simulink model "s1"  (Simulink 2.00)
settings: Solver=ode113  StartTime=0.0  StopTime=tstop  MaxStep=1e-3  RelTol=1e-6  AbsTol=1e-5
values from neighbouring files (symbols this model uses):
  Domega = 0    [P1HP.M]    (also in PSPH.M)
  H = J*wbm*wbm/(2*Sb)    (= 2.36870505626)    [P1HP.M]    (also in PSPH.M = 1.39074103839)
  Psidso = 0    [M1.M]    (also in M4.M; M4STP.M; M5.M)
  Psipdro = 0    [M1.M]    (also in M4.M; M4STP.M; M5.M; M6.M)
  Psipqro = 0    [M1.M]    (also in M4.M = Vm; M4STP.M = Vm; M5.M; M6.M)
  Psiqso = 0    [M1.M]    (also in M4.M = Vm; M4STP.M = Vm; M5.M; M6.M)
  rpr = 1.99    [P1HP.M]    (also in PSPH.M = 4.12)
  rs = 3.35    [P1HP.M]
  Tfactor = (3*P)/(4*wb)    (= 0.00795774715459)    [P1HP.M]    (also in PSPH.M = 0.00530516476973)
  tmech_time = [0 0.8 0.8 1.2 1.2 1.6 1.6 tstop]    [M1.M]    (also in M6.M = [0 1.5 1.5 1.75 1.75 2.0 2.0 2.25 2.25 2.5])
  tmech_value = [0 0 -0.5 -0.5 -1. -1. -0.5 -0.5]*Tb    [M1.M]    (also in M6.M = [0 0 -Tb -Tb -Tb/2 -Tb/2 -Tb -Tb 0 0 ])
  Vm = Vrated*sqrt(2/3)    [M4.M]    (also in P1HP.M; PSPH.M = Vrated*sqrt(2))
  wb = 2*pi*frated    (= 376.991118431)    [P1HP.M]    (also in PSPH.M)
  wrbywbo = 0    [M1.M]    (also in M4.M = 1; M4STP.M = 1; M5.M; M6.M)
  xls = 6.94e-3*wb    (= 2.61631836191)    [P1HP.M]
  xM = 1/(1/xm + 1/xls + 1/xplr)    (= 1.2810101836)    [P1HP.M]
  xplr = xls    (= 2.61631836191)    [P1HP.M]    (also in PSPH.M = 2.12)
  Zb = Vrated*Vrated/Sb    (= 53.3333333333)    [P1HP.M]    (also in PSPH.M = 64.8793565684)
settings Model: MaxOrder=4  SaveTime=off  SaveOutput=off  ConsistencyChecking=off

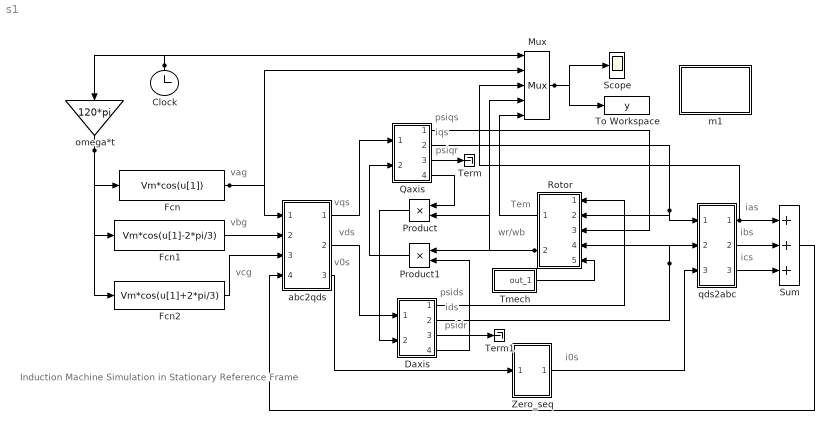
== system s1 ==
  note: Induction Machine Simulation
      |   in Stationary Reference Frame
  note: i0s
  note: vqs
  note: Tem
  note: wr/wb
  note: vag
  note: vcg
  note: vbg
  note: v0s
  note: psiqs
  note: iqs
  note: psiqr
  note: ibs
  note: ics
  note: vds
  note: psids
  note: ids
  note: psidr
  note: ias
  Clock : Clock
      settings: Orientation=up  DeleteFcn=simclock BlockIsBeingDestroyed  PostSaveFcn=simclock Save
  Daxis : Subsystem
  Fcn : Fcn  Expr=Vm*cos(u[1])
  Fcn1 : Fcn  Expr=Vm*cos(u[1]-2*pi/3)
  Fcn2 : Fcn  Expr=Vm*cos(u[1]+2*pi/3)
  m1 : Subsystem
      settings: OpenFcn=m1
      mask Type: Masked block of m1.m
      mask Help: Uses m1.m to initialize and plot
      mask Display: disp('Initialize\nand plot')
  Mux : Mux  Inputs=5
  Product : Product  Orientation=left  Inputs=2
  Product1 : Product  Orientation=left  Inputs=2
  Qaxis : Subsystem
  Rotor : Subsystem  Orientation=left
  Scope : Scope
      settings: TickLabels=on  TimeRange=2  YMin=-30  YMax=30  SaveToWorkspace=off  SaveName=ScopeData  LimitMaxRows=off  Decimation=2
  Sum : Sum  Inputs=+++
  Term : Terminator
  Term1 : Terminator
  Tmech : Subsystem  mask(Repeating table){rep_seq_t=tmech_time, rep_seq_y=tmech_value}
      mask prompts: rep_seq_t "Time values:"; rep_seq_y "Output values:"
      mask help: Repeating table.
      mask init:
      | period = max(rep_seq_t);
      mask Help: Repeats cycle given in table. Time values should be monotonically increasing.
      mask Display: plot([rep_seq_t,rep_seq_t+period,rep_seq_t+2*period,rep_seq_t(1)+3*period],[rep_seq_y,rep_seq_y,rep_seq_y,rep_seq_y(1)])
  To Workspace : ToWorkspace  VariableName=y  SampleTime=0
      settings: Buffer=80000
  Zero_seq : Subsystem
  abc2qds : Subsystem
  omega*t : Gain  Orientation=down  Gain=120*pi
  qds2abc : Subsystem
  wires:
  Daxis/2(out_ids) -> qds2abc/2(in_ids), Rotor/4(in_ids)
  Product1/1 -> Qaxis/2(in_(wr/wb)*psidr')
  Qaxis/1(out_psiqs) -> Rotor/3(in_psiqs)
  abc2qds/2(out_vds) -> Daxis/1(in_vds)
  abc2qds/1(out_vqs) -> Qaxis/1(in_vqs)
  Qaxis/2(out_iqs) -> qds2abc/1(in_iqs), Rotor/2(in_iqs)
  Product/1 -> Daxis/2(in_(wr/wb)*psiqr')
  Rotor/2(out_wr/wb) -> Product/2, Product1/1, Mux/4
  Mux/1 -> To Workspace/1, Scope/1
  Rotor/1(out_Tem) -> Mux/5
  omega*t/1 -> Fcn/1, Fcn1/1, Fcn2/1
  Fcn1/1 -> abc2qds/2(in_vbg)
  Clock/1 -> omega*t/1, Mux/1
  Fcn/1 -> abc2qds/1(in_vag), Mux/2
  Qaxis/4(out_psiqr') -> Product/1
  Daxis/4(out_psidr') -> Product1/2
  abc2qds/3(out_v0s) -> Zero_seq/1(in_v0s)
  qds2abc/2(out_ibs) -> Sum/2
  qds2abc/3(out_ics) -> Sum/3
  Zero_seq/1(out_i0s) -> qds2abc/3(in_i0s)
  qds2abc/1(out_ias) -> Sum/1, Mux/3
  Sum/1 -> abc2qds/4(ias+ibs+ics)
  Fcn2/1 -> abc2qds/3(in_vcg)
  Qaxis/3(out_iqr') -> Term/1
  Daxis/3(out_idr') -> Term1/1
  Daxis/1(out_psids) -> Rotor/1(in_psids)
  Tmech/1(out_1) -> Rotor/5(in_Tmech)

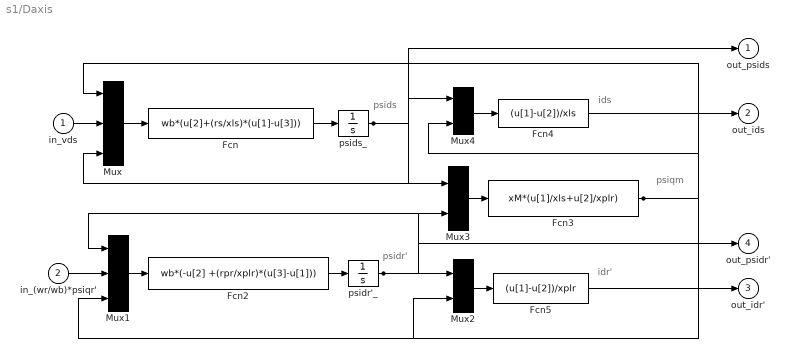
== system s1/Daxis ==
  note: ids
  note: psids
  note: psiqm
  note: idr'
  note: psidr'
  in_vds : Inport  Port=1  PortWidth=-1  SampleTime=-1
  in_(wr/wb)*psiqr' : Inport  Port=2  PortWidth=-1  SampleTime=-1
  Fcn : Fcn  Expr=wb*(u[2]+(rs/xls)*(u[1]-u[3]))
  Fcn2 : Fcn  Expr=wb*(-u[2] +(rpr/xplr)*(u[3]-u[1]))
  Fcn3 : Fcn  Expr=xM*(u[1]/xls+u[2]/xplr)
  Fcn4 : Fcn  Expr=(u[1]-u[2])/xls
  Fcn5 : Fcn  Expr=(u[1]-u[2])/xplr
  Mux : Mux  Inputs=3
  Mux1 : Mux  Inputs=3
  Mux2 : Mux  Inputs=2
  Mux3 : Mux  Inputs=2
  Mux4 : Mux  Inputs=2
  psidr'_ : Integrator  ExternalReset=none  InitialConditionSource=internal  InitialCondition=Psipdro  LimitOutput=off  UpperSaturationLimit=inf  LowerSaturationLimit=-inf  ShowSaturationPort=off  ShowStatePort=off  AbsoluteTolerance=auto
  psids_ : Integrator  ExternalReset=none  InitialConditionSource=internal  InitialCondition=Psidso  LimitOutput=off  UpperSaturationLimit=inf  LowerSaturationLimit=-inf  ShowSaturationPort=off  ShowStatePort=off  AbsoluteTolerance=auto
  out_psids : Outport  Port=1  InitialOutput=0
  out_ids : Outport  Port=2  InitialOutput=0
  out_idr' : Outport  Port=3  InitialOutput=0
  out_psidr' : Outport  Port=4  InitialOutput=0
  wires:
  Mux2/1 -> Fcn5/1
  psidr'_/1 -> Mux2/1, Mux3/2, Mux1/1, out_psidr'/1
  Mux1/1 -> Fcn2/1
  Fcn3/1 -> Mux2/2, Mux/1, Mux1/3, Mux4/2
  psids_/1 -> Mux/3, Mux4/1, Mux3/1, out_psids/1
  Mux4/1 -> Fcn4/1
  Mux3/1 -> Fcn3/1
  Fcn2/1 -> psidr'_/1
  Fcn/1 -> psids_/1
  Mux/1 -> Fcn/1
  Fcn4/1 -> out_ids/1
  in_vds/1 -> Mux/2
  in_(wr/wb)*psiqr'/1 -> Mux1/2
  Fcn5/1 -> out_idr'/1

== system s1/m1 ==
  note: Masked block of m1.m to initialize s1.m
      | and plot results

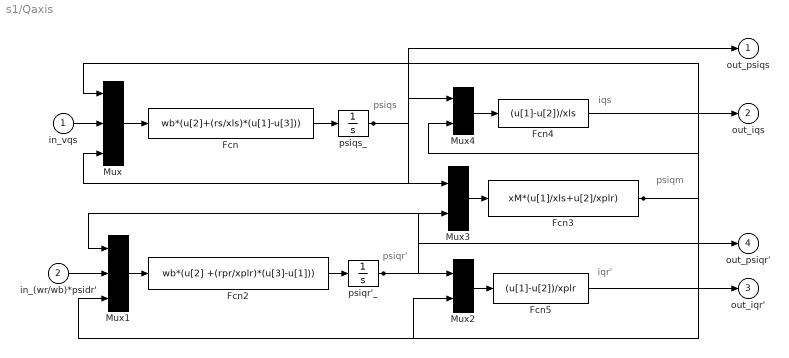
== system s1/Qaxis ==
  note: iqs
  note: psiqs
  note: psiqm
  note: iqr'
  note: psiqr'
  in_vqs : Inport  Port=1  PortWidth=-1  SampleTime=-1
  in_(wr/wb)*psidr' : Inport  Port=2  PortWidth=-1  SampleTime=-1
  Fcn : Fcn  Expr=wb*(u[2]+(rs/xls)*(u[1]-u[3]))
  Fcn2 : Fcn  Expr=wb*(u[2] +(rpr/xplr)*(u[3]-u[1]))
  Fcn3 : Fcn  Expr=xM*(u[1]/xls+u[2]/xplr)
  Fcn4 : Fcn  Expr=(u[1]-u[2])/xls
  Fcn5 : Fcn  Expr=(u[1]-u[2])/xplr
  Mux : Mux  Inputs=3
  Mux1 : Mux  Inputs=3
  Mux2 : Mux  Inputs=2
  Mux3 : Mux  Inputs=2
  Mux4 : Mux  Inputs=2
  psiqr'_ : Integrator  ExternalReset=none  InitialConditionSource=internal  InitialCondition=Psipqro  LimitOutput=off  UpperSaturationLimit=inf  LowerSaturationLimit=-inf  ShowSaturationPort=off  ShowStatePort=off  AbsoluteTolerance=auto
  psiqs_ : Integrator  ExternalReset=none  InitialConditionSource=internal  InitialCondition=Psiqso  LimitOutput=off  UpperSaturationLimit=inf  LowerSaturationLimit=-inf  ShowSaturationPort=off  ShowStatePort=off  AbsoluteTolerance=auto
  out_psiqs : Outport  Port=1  InitialOutput=0
  out_iqs : Outport  Port=2  InitialOutput=0
  out_iqr' : Outport  Port=3  InitialOutput=0
  out_psiqr' : Outport  Port=4  InitialOutput=0
  wires:
  Mux2/1 -> Fcn5/1
  psiqr'_/1 -> Mux2/1, Mux3/2, Mux1/1, out_psiqr'/1
  Mux1/1 -> Fcn2/1
  Fcn3/1 -> Mux2/2, Mux/1, Mux1/3, Mux4/2
  psiqs_/1 -> Mux/3, Mux4/1, Mux3/1, out_psiqs/1
  Mux4/1 -> Fcn4/1
  Mux3/1 -> Fcn3/1
  Fcn2/1 -> psiqr'_/1
  Fcn/1 -> psiqs_/1
  Mux/1 -> Fcn/1
  Fcn4/1 -> out_iqs/1
  in_vqs/1 -> Mux/2
  in_(wr/wb)*psidr'/1 -> Mux1/2
  Fcn5/1 -> out_iqr'/1

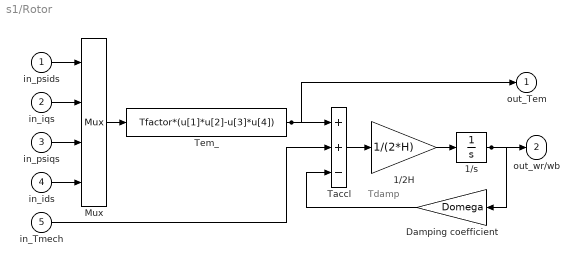
== system s1/Rotor ==
  note: Tdamp
  in_psids : Inport  Port=1  PortWidth=-1  SampleTime=-1
  in_iqs : Inport  Port=2  PortWidth=-1  SampleTime=-1
  in_psiqs : Inport  Port=3  PortWidth=-1  SampleTime=-1
  in_ids : Inport  Port=4  PortWidth=-1  SampleTime=-1
  in_Tmech : Inport  Port=5  PortWidth=-1  SampleTime=-1
  1/2H : Gain  Gain=1/(2*H)
  1/s : Integrator  ExternalReset=none  InitialConditionSource=internal  InitialCondition=wrbywbo  LimitOutput=off  UpperSaturationLimit=inf  LowerSaturationLimit=-inf  ShowSaturationPort=off  ShowStatePort=off  AbsoluteTolerance=auto
  Damping coefficient : Gain  Orientation=left  Gain=Domega
  Mux : Mux  Inputs=4
  Taccl : Sum  Inputs=++-
  Tem_ : Fcn  Expr=Tfactor*(u[1]*u[2]-u[3]*u[4])
  out_Tem : Outport  Port=1  InitialOutput=0
  out_wr/wb : Outport  Port=2  InitialOutput=0
  wires:
  in_Tmech/1 -> Taccl/2
  Taccl/1 -> 1/2H/1
  1/2H/1 -> 1/s/1
  Tem_/1 -> Taccl/1, out_Tem/1
  1/s/1 -> out_wr/wb/1, Damping coefficient/1
  Damping coefficient/1 -> Taccl/3
  Mux/1 -> Tem_/1
  in_psids/1 -> Mux/1
  in_iqs/1 -> Mux/2
  in_psiqs/1 -> Mux/3
  in_ids/1 -> Mux/4

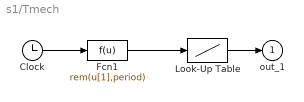
== system s1/Tmech ==
  Clock : Clock
      settings: DeleteFcn=simclock BlockIsBeingDestroyed  PostSaveFcn=simclock Save
  Fcn1 : Fcn  Expr=rem(u[1],period)
  Look-Up Table : Lookup  InputValues=rep_seq_t  OutputValues=rep_seq_y
  out_1 : Outport  Port=1  InitialOutput=0
  wires:
  Look-Up Table/1 -> out_1/1
  Clock/1 -> Fcn1/1
  Fcn1/1 -> Look-Up Table/1

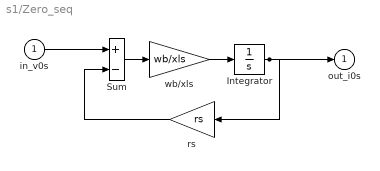
== system s1/Zero_seq ==
  in_v0s : Inport  Port=1  PortWidth=-1  SampleTime=-1
  Integrator : Integrator  ExternalReset=none  InitialConditionSource=internal  InitialCondition=0  LimitOutput=off  UpperSaturationLimit=inf  LowerSaturationLimit=-inf  ShowSaturationPort=off  ShowStatePort=off  AbsoluteTolerance=auto
  Sum : Sum  Inputs=+-
  rs : Gain  Orientation=left  Gain=rs
  wb/xls : Gain  Gain=wb/xls
  out_i0s : Outport  Port=1  InitialOutput=0
  wires:
  rs/1 -> Sum/2
  Sum/1 -> wb/xls/1
  wb/xls/1 -> Integrator/1
  in_v0s/1 -> Sum/1
  Integrator/1 -> rs/1, out_i0s/1

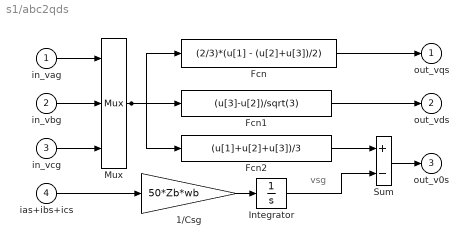
== system s1/abc2qds ==
  note: vsg
  in_vag : Inport  Port=1  PortWidth=-1  SampleTime=-1
  in_vbg : Inport  Port=2  PortWidth=-1  SampleTime=-1
  in_vcg : Inport  Port=3  PortWidth=-1  SampleTime=-1
  ias+ibs+ics : Inport  Port=4  PortWidth=-1  SampleTime=-1
  1/Csg : Gain  Gain=50*Zb*wb
  Fcn : Fcn  Expr=(2/3)*(u[1] - (u[2]+u[3])/2)
  Fcn1 : Fcn  Expr=(u[3]-u[2])/sqrt(3)
  Fcn2 : Fcn  Expr=(u[1]+u[2]+u[3])/3
  Integrator : Integrator  ExternalReset=none  InitialConditionSource=internal  InitialCondition=0  LimitOutput=off  UpperSaturationLimit=inf  LowerSaturationLimit=-inf  ShowSaturationPort=off  ShowStatePort=off  AbsoluteTolerance=auto
  Mux : Mux  Inputs=3
  Sum : Sum  Inputs=+-
  out_vqs : Outport  Port=1  InitialOutput=0
  out_vds : Outport  Port=2  InitialOutput=0
  out_v0s : Outport  Port=3  InitialOutput=0
  wires:
  in_vag/1 -> Mux/1
  in_vbg/1 -> Mux/2
  in_vcg/1 -> Mux/3
  Fcn/1 -> out_vqs/1
  Mux/1 -> Fcn1/1, Fcn/1, Fcn2/1
  Fcn1/1 -> out_vds/1
  Sum/1 -> out_v0s/1
  Fcn2/1 -> Sum/1
  1/Csg/1 -> Integrator/1
  ias+ibs+ics/1 -> 1/Csg/1
  Integrator/1 -> Sum/2

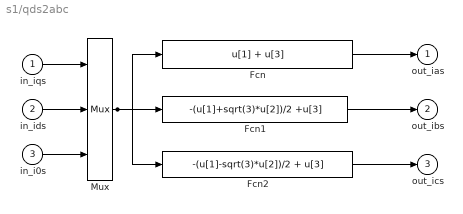
== system s1/qds2abc ==
  in_iqs : Inport  Port=1  PortWidth=-1  SampleTime=-1
  in_ids : Inport  Port=2  PortWidth=-1  SampleTime=-1
  in_i0s : Inport  Port=3  PortWidth=-1  SampleTime=-1
  Fcn : Fcn  Expr=u[1] + u[3]
  Fcn1 : Fcn  Expr=-(u[1]+sqrt(3)*u[2])/2 +u[3]
  Fcn2 : Fcn  Expr=-(u[1]-sqrt(3)*u[2])/2 + u[3]
  Mux : Mux  Inputs=3
  out_ias : Outport  Port=1  InitialOutput=0
  out_ibs : Outport  Port=2  InitialOutput=0
  out_ics : Outport  Port=3  InitialOutput=0
  wires:
  in_ids/1 -> Mux/2
  in_iqs/1 -> Mux/1
  in_i0s/1 -> Mux/3
  Fcn1/1 -> out_ibs/1
  Fcn/1 -> out_ias/1
  Mux/1 -> Fcn1/1, Fcn/1, Fcn2/1
  Fcn2/1 -> out_ics/1
